simulink model "understandingof_secwave"  (R2024b)
settings: Solver=VariableStepAuto  StartTime=0.0  StopTime=10.0  MaxStep=0.001  RelTol=1e-3
settings Model: Creator=admin  LastModifiedBy=admin

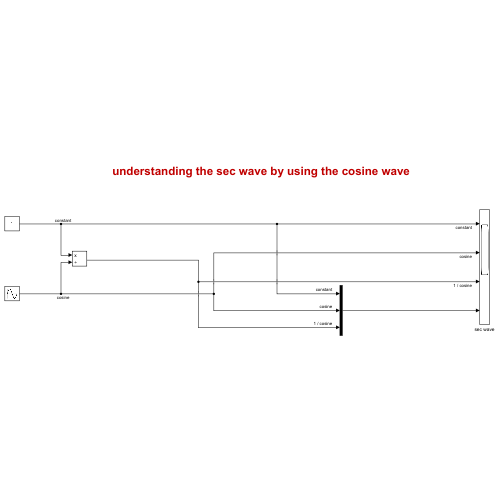
[thumbnail: Simulink's stored preview of the top-level diagram]
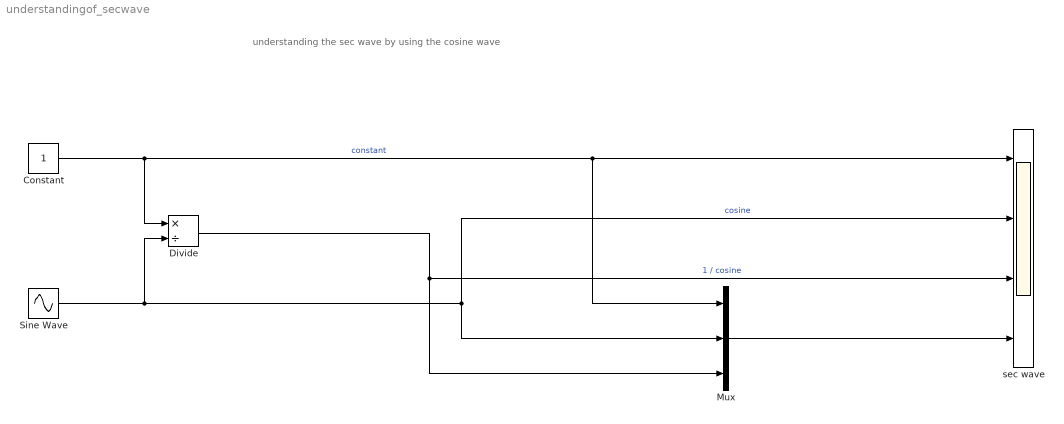
== system understandingof_secwave ==
  note: understanding the sec wave by using the cosine wave
  Constant : Constant
  Divide : Product  Inputs=*/
  Mux : Mux  Inputs=3
  Sine Wave : Sin  Phase=pi/2  SampleTime=0
  sec wave : Scope  NumInputPorts=4
  wires:
  Constant/1 -> Mux/1, sec wave/1, Divide/1  "constant"
  Divide/1 -> sec wave/3, Mux/3  "1 / cosine"
  Mux/1 -> sec wave/4
  Sine Wave/1 -> sec wave/2, Mux/2, Divide/2  "cosine"
